simulink model "untitled"  (R2025b)
settings: Solver=VariableStepAuto  StartTime=0.0  StopTime=10.0  RelTol=1e-3
settings Model: Creator=Liam  LastModifiedBy=Liam

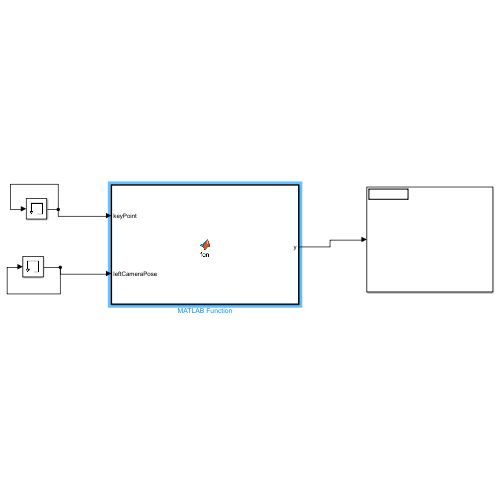
[thumbnail: Simulink's stored preview of the top-level diagram]
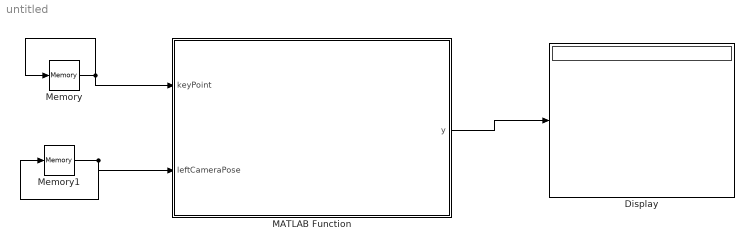
== system untitled ==
  Display : Display
  MATLAB Function : MATLAB Function  TreatAsAtomicUnit=on
  Memory : Memory  InitialCondition=[100 100 100]
  Memory1 : Memory  InitialCondition=[100 100 100 0 0 0]
  wires:
  Memory/1 -> Memory/1, MATLAB Function/1(keyPoint)
  MATLAB Function/1(y) -> Display/1
  Memory1/1 -> MATLAB Function/2(leftCameraPose), Memory1/1

== matlab function untitled/MATLAB Function ==
  data: y output; keyPoint input; leftCameraPose input; stereoParams data_store_memory
function y = fcn(keyPoint, leftCameraPose)
p = zeros(4);
p(1:3) = keyPoint(1:3);
p(4) = 1;
y = getWorldToImage(p, leftCameraPose, stereoParams);
